simulink model "sbm65_kin"  (R2016b)
settings: Solver=ode45  StartTime=0.0  StopTime=150  MaxStep=.01  RelTol=1e-6  EnableMultiTasking=on
values from neighbouring files (symbols this model uses):
  angFormation1 = 0    [start.m]
  angFormation2 = deg2rad(-45)    [start.m]
  angFormation3 = deg2rad(45)    [start.m]
  deg = pi/180    (= 0.0174532925199)    [db_droni.m]    (also in temp.mat; tslip1.m)
  Di = -77    [start.m]    (also in temp.mat = -77.0888961142)
  ka = 5    [start.m]
  kb = (2/pi*kp - ka + 0.1)*3/5    (= -2.74901406829)    [start.m]
  kp = 0.5    [start.m]
  mis = [  50,   0,   0,  10 ... (first row only)    [start.m]    (also in tslip1.m = [0 0 0)
  wind =     [temp.mat]
  X =     [temp.mat]    (also in tslip1.m = [X [u;eig(AB(1:2,1:2))]])
  X6_ini1 = [2 0   0 0 0 0]'    [start.m]
  X6_ini2 = [  0   0   0 0 0 0]'    [start.m]
  X6_ini3 = [  0  0   0 0 0 0]'    [start.m]
  X7_ini1 = [40 0 -77 1 0 0 0]'    [start.m]
  X7_ini2 = [30 -10 -77 1 0 0 0]'    [start.m]
  X7_ini3 = [20 10 -77 1 0 0 0]'    [start.m]
  xmax = 115    [start.m]
  xmin = -150    [start.m]
  ymax = 105    [start.m]
  ymin = -120    [start.m]
undefined symbols (not defined in the file or in its folder): magnitude, sfunxy2
libraries: simulink x3
settings Model: Creator=hdsvieira  LastModifiedBy=Pedro
settings SolverCC: MaxOrder=2
settings DataIOCC: LimitDataPoints=on  SaveFormat=Array  SignalLoggingSaveFormat=ModelDataLogs  SaveOutput=off  SaveTime=off  SignalLoggingName=sigsOut
settings OptimizationCC: LifeSpan=inf
settings DebuggingCC: ReadBeforeWriteMsg=DisableAll  WriteAfterWriteMsg=DisableAll  WriteAfterReadMsg=DisableAll  SaveWithParameterizedLinksMsg=none  MultiTaskDSMMsg=none  MultiTaskCondExecSysMsg=none  SFUnexpectedBacktrackingDiag=warning  SFNoUnconditionalDefaultTransitionDiag=warning  SFExecutionAtInitializationDiag=none
settings HardwareCC: ProdBitPerPointer=32  ProdBitPerSizeT=32  ProdBitPerPtrDiffT=32  ProdLargestAtomicFloat=None  ProdIntDivRoundTo=Undefined  ProdEndianess=Unspecified  ProdWordSize=32  ProdHWDeviceType=32-bit Generic  TargetUnknown=on
settings ModelReferenceCC: UpdateModelReferenceTargets=IfOutOfDate  PropagateSignalLabelsOutOfModel=off
settings SFSimCC: SFSimEcho=off
settings GRTTargetCC: TargetLangStandard=C89/C90 (ANSI)  GeneratePreprocessorConditionals=Disable all  CombineOutputUpdateFcns=off  GRTInterface=on
settings ConfigComp: CovMetricSettings=dw  CovHtmlReporting=on  CovSaveCumulativeToWorkspaceVar=on  CovSaveSingleToWorkspaceVar=on  CovExternalEMLEnable=off

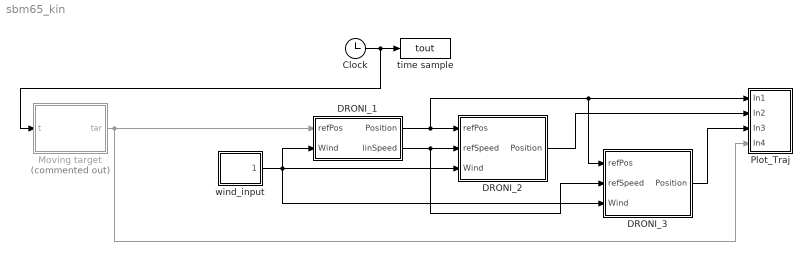
== system sbm65_kin ==
  Clock : Clock
  DRONI_1 : Subsystem
  DRONI_2 : Subsystem
  DRONI_3 : Subsystem
  Moving target : MATLAB Function  Commented=on  TreatAsAtomicUnit=on
  Plot_Traj : Subsystem  LoadFcn=sfunxy2([],[],[],'LoadBlock')  StartFcn=sfunxy2([],[],[],'Start')  StopFcn=sfunxy2([],[],[],'Stop')
      settings: CopyFcn=sfunxy2([],[],[],'CopyBlock')  DeleteFcn=sfunxy2([],[],[],'DeleteBlock')  NameChangeFcn=sfunxy2([],[],[],'NameChange')
  time sample : ToWorkspace  VariableName=tout  SampleTime=X.Toutput
      settings: MaxDataPoints=5000
  wind_input : Subsystem
  wires:
  Clock/1 -> time sample/1, Moving target/1(t)
  DRONI_1/2(linSpeed) -> DRONI_3/2(refSpeed), DRONI_2/2(refSpeed)
  DRONI_3/1(Position) -> Plot_Traj/3(In3)
  DRONI_2/1(Position) -> Plot_Traj/2(In2)
  DRONI_1/1(Position) -> DRONI_3/1(refPos), Plot_Traj/1(In1), DRONI_2/1(refPos)
  Moving target/1(tar) -> DRONI_1/1(refPos), Plot_Traj/4(In4)
  wind_input/1(U_wind) -> DRONI_3/3(Wind), DRONI_1/2(Wind), DRONI_2/3(Wind)

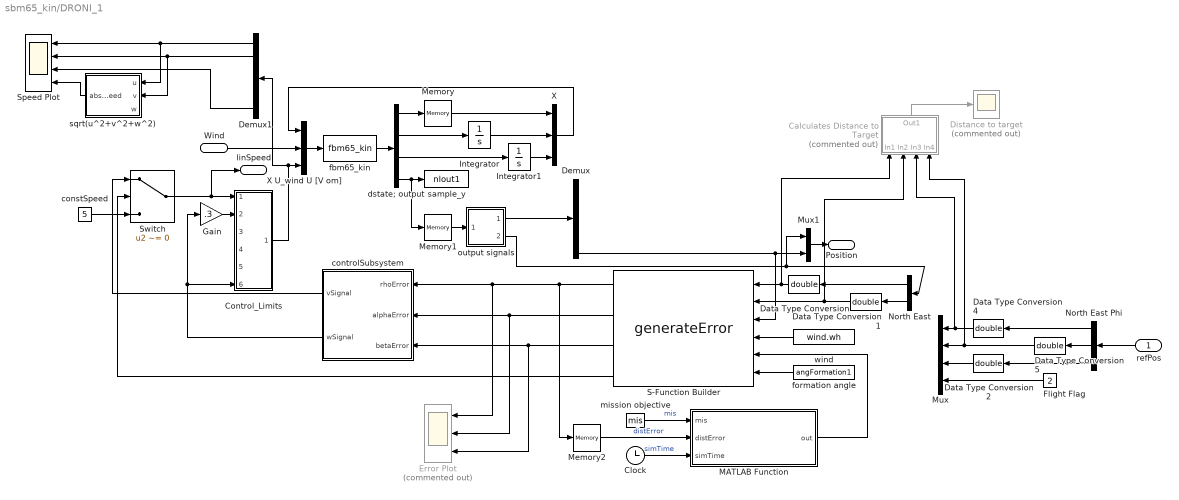
== system sbm65_kin/DRONI_1 ==
  refPos : Inport
  Wind : Inport  Port=2
  Calculates Distance to Target : Subsystem  Commented=on
  Clock : Clock
  Control_Limits : Subsystem
  Data Type Conversion{,1..2,4..5} (5 alike) : DataTypeConversion  DisableCoverage=on  OutDataTypeStr=double
  Demux : Demux  Outputs=5
  Demux1 : Demux  Outputs=6
  Distance to target : Scope  Commented=on
  Error Plot : Scope  Commented=on  NumInputPorts=3
  Flight Flag : Constant  Value=2
  Gain : Gain  Gain=.3
  Integrator : Integrator  InitialCondition=X7_ini1
  Integrator1 : Integrator  InitialCondition=zeros(1,8)
  MATLAB Function : MATLAB Function  TreatAsAtomicUnit=on
  Memory : Memory  X0=X6_ini1
  Memory1 : Memory  X0=zeros(22,1)
  Memory2 : Memory  X0=10
  Mux : Mux
  Mux1 : Mux  Inputs=2
  North East : Demux  Outputs=[1 1]
  North East Phi : Demux  Outputs=[1 1 1]
  S-Function Builder : S-Function  InitFcn=try, set_param(gcb,'FunctionName','generateError'), end  FunctionName=generateError  SFunctionModules=generateError_wrapper  SFunctionDeploymentMode=off  EnableBusSupport=off  mask(S-Function Builder){}
      mask help: Simulink:masks:SFunctionBuilder_MD
      mask init:
      | val = [[.9  0.75 0.75 1 1 .9 .9 1]',[1 1 0.75 0.75 .9 .9 1 .9]'];try , sys = get_param(gcb,'SfunBuilderFcnName');if isempty(sys), sys = get_param(gcb,'FunctionName'); end,catch, sys = get_param(gcb,'FunctionName'); end
      settings: CopyFcn=set_param(gcbh,'LinkStatus','none')  PreSaveFcn=try, set_param(gcb,'FunctionName','generateError'), end  OpenFcn=sfunctionwizard(gcbh)
      mask Display: plot(val(:,1),val(:,2)),disp(sys), port_label('input',1,'y0'), port_label('input',2,'x0'), port_label('input',3,'theta0'), port_label('input',4,'wind'), port_label('input',5,'objective'), port_label('input',6,'angOffset'), port_label('output',1,'rho'), port_label('output',2,'alpha'), port_label('output',3,'beta'), port_label('output',4,'flightMode')
  Speed Plot : Scope  NumInputPorts=4
  Switch : Switch  Criteria=u2 ~= 0  Threshold=.5
  X : Mux  Inputs=[6 7 8]
  X U_wind U [V om] : Mux  Inputs=[21 5 6]
  constSpeed : Constant  Value=5
  controlSubsystem : Subsystem
  dstate; output : Demux  Outputs="[6 7  8  22]"
  fbm65_kin : MATLABFcn  MATLABFcn=fbm65_kin  OutputDimensions=43
  formation angle : Constant  Value=angFormation1
  mission objective : Constant  Value=mis
  output signals : Subsystem
  sample_y : ToWorkspace  VariableName=nlout1  SampleTime=X.Toutput
      settings: MaxDataPoints=5000
  sqrt(u^2+v^2+w^2) : Subsystem
  wind : Constant  Value=wind.wh
  Position : Outport
  linSpeed : Outport  Port=2
  wires:
  North East/2 -> Data Type Conversion1/1
  Memory1/1 -> output signals/1(nlout)
  X U_wind U [V om]/1 -> fbm65_kin/1
  fbm65_kin/1 -> dstate; output/1
  Control_Limits/1(Out1) -> Demux1/1, X U_wind U [V om]/3
  dstate; output/3 -> Integrator1/1
  Integrator/1 -> X/2
  wind/1 -> S-Function Builder/4
  Integrator1/1 -> X/3
  dstate; output/1 -> Memory/1
  Memory/1 -> X/1
  Data Type Conversion/1 -> S-Function Builder/1, Calculates Distance to Target/1(In1)
  North East/1 -> Data Type Conversion/1
  dstate; output/2 -> Integrator/1
  output signals/1(Out1) -> Demux/1
  X/1 -> X U_wind U [V om]/1
  Data Type Conversion1/1 -> S-Function Builder/2, Calculates Distance to Target/2(In2)
  Wind/1 -> X U_wind U [V om]/2
  controlSubsystem/2(wSignal) -> Control_Limits/6(In6), Gain/1
  Switch/1 -> linSpeed/1, Control_Limits/1(In1)
  S-Function Builder/4 -> Switch/2
  constSpeed/1 -> Switch/3
  controlSubsystem/1(vSignal) -> Switch/1
  dstate; output/4 -> sample_y/1, Memory1/1
  Demux/5 -> Mux1/2, S-Function Builder/3
  output signals/2(Out2) -> Mux1/1, North East/1
  S-Function Builder/1 -> Memory2/1, Error Plot/1, controlSubsystem/1(rhoError)
  S-Function Builder/2 -> Error Plot/2, controlSubsystem/2(alphaError)
  S-Function Builder/3 -> Error Plot/3, controlSubsystem/3(betaError)
  Clock/1 -> MATLAB Function/3(simTime)  "simTime"
  Memory2/1 -> MATLAB Function/2(distError)  "distError"
  mission objective/1 -> MATLAB Function/1(mis)  "mis"
  Demux1/1 -> Speed Plot/1, sqrt(u^2+v^2+w^2)/1(u)
  Demux1/2 -> sqrt(u^2+v^2+w^2)/2(v), Speed Plot/2
  sqrt(u^2+v^2+w^2)/1(abs speed) -> Speed Plot/4
  Gain/1 -> Control_Limits/2(In2)
  North East Phi/2 -> Data Type Conversion5/1
  North East Phi/1 -> Data Type Conversion4/1
  refPos/1 -> North East Phi/1
  North East Phi/3 -> Data Type Conversion2/1
  Data Type Conversion4/1 -> Calculates Distance to Target/3(In3), Mux/1
  Data Type Conversion5/1 -> Calculates Distance to Target/4(In4), Mux/2
  Data Type Conversion2/1 -> Mux/3
  Flight Flag/1 -> Mux/4
  formation angle/1 -> S-Function Builder/6
  Mux1/1 -> Position/1
  Demux1/6 -> Speed Plot/3
  Calculates Distance to Target/1(Out1) -> Distance to target/1
  MATLAB Function/1(out) -> S-Function Builder/5

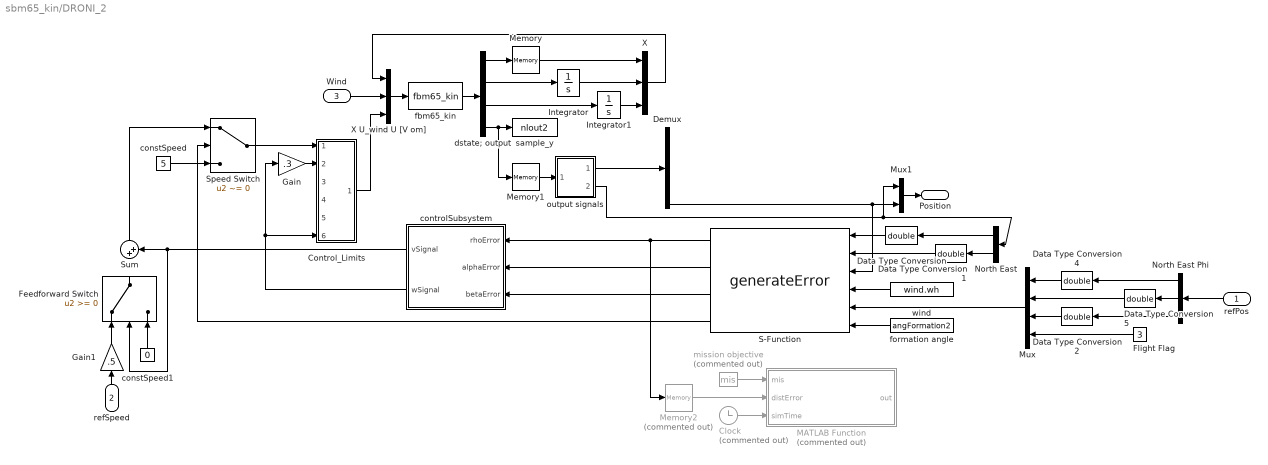
== system sbm65_kin/DRONI_2 ==
  refPos : Inport
  refSpeed : Inport  Port=2
  Wind : Inport  Port=3
  Clock : Clock  Commented=on
  Control_Limits : Subsystem
  Data Type Conversion{,1..2,4..5} (5 alike) : DataTypeConversion  DisableCoverage=on  OutDataTypeStr=double
  Demux : Demux  Outputs=5
  Feedforward Switch : Switch
  Flight Flag : Constant  Value=3
  Gain : Gain  Gain=.3
  Gain1 : Gain  Gain=.5
  Integrator : Integrator  InitialCondition=X7_ini2
  Integrator1 : Integrator  InitialCondition=zeros(1,8)
  MATLAB Function : MATLAB Function  Commented=on  TreatAsAtomicUnit=on
  Memory : Memory  X0=X6_ini2
  Memory1 : Memory  X0=zeros(22,1)
  Memory2 : Memory  Commented=on  X0=10
  Mux : Mux
  Mux1 : Mux  Inputs=2
  North East : Demux  Outputs=[1 1]
  North East Phi : Demux  Outputs=[1 1 1]
  S-Function : S-Function  FunctionName=generateError  SFunctionDeploymentMode=off  EnableBusSupport=off
  Speed Switch : Switch  Criteria=u2 ~= 0  Threshold=.5
  Sum : Sum  Inputs=|++
  X : Mux  Inputs=[6 7 8]
  X U_wind U [V om] : Mux  Inputs=[21 5 6]
  constSpeed : Constant  Value=5
  constSpeed1 : Constant  Value=0
  controlSubsystem : Subsystem
  dstate; output : Demux  Outputs="[6 7  8  22]"
  fbm65_kin : MATLABFcn  MATLABFcn=fbm65_kin  OutputDimensions=43
  formation angle : Constant  Value=angFormation2
  mission objective : Constant  Commented=on  Value=mis
  output signals : Subsystem
  sample_y : ToWorkspace  VariableName=nlout2  SampleTime=X.Toutput
      settings: MaxDataPoints=5000
  wind : Constant  Value=wind.wh
  Position : Outport
  wires:
  North East/2 -> Data Type Conversion1/1
  Memory1/1 -> output signals/1(nlout)
  X U_wind U [V om]/1 -> fbm65_kin/1
  fbm65_kin/1 -> dstate; output/1
  Control_Limits/1(Out1) -> X U_wind U [V om]/3
  dstate; output/3 -> Integrator1/1
  Integrator/1 -> X/2
  wind/1 -> S-Function/4
  Integrator1/1 -> X/3
  dstate; output/1 -> Memory/1
  Memory/1 -> X/1
  Data Type Conversion/1 -> S-Function/1
  North East/1 -> Data Type Conversion/1
  dstate; output/2 -> Integrator/1
  output signals/1(Out1) -> Demux/1
  X/1 -> X U_wind U [V om]/1
  Data Type Conversion1/1 -> S-Function/2
  Wind/1 -> X U_wind U [V om]/2
  mission objective/1 -> MATLAB Function/1(mis)
  Clock/1 -> MATLAB Function/3(simTime)
  Memory2/1 -> MATLAB Function/2(distError)
  Speed Switch/1 -> Control_Limits/1(In1)
  S-Function/4 -> Speed Switch/2
  constSpeed/1 -> Speed Switch/3
  controlSubsystem/1(vSignal) -> Feedforward Switch/2, Sum/2
  dstate; output/4 -> sample_y/1, Memory1/1
  Demux/5 -> Mux1/2, S-Function/3
  output signals/2(Out2) -> Mux1/1, North East/1
  S-Function/1 -> Memory2/1, controlSubsystem/1(rhoError)
  S-Function/2 -> controlSubsystem/2(alphaError)
  S-Function/3 -> controlSubsystem/3(betaError)
  Data Type Conversion4/1 -> Mux/1
  Data Type Conversion5/1 -> Mux/2
  Data Type Conversion2/1 -> Mux/3
  Mux/1 -> S-Function/5
  Flight Flag/1 -> Mux/4
  formation angle/1 -> S-Function/6
  Sum/1 -> Speed Switch/1
  controlSubsystem/2(wSignal) -> Control_Limits/6(In6), Gain/1
  refSpeed/1 -> Gain1/1
  Gain/1 -> Control_Limits/2(In2)
  North East Phi/2 -> Data Type Conversion5/1
  North East Phi/1 -> Data Type Conversion4/1
  refPos/1 -> North East Phi/1
  North East Phi/3 -> Data Type Conversion2/1
  Mux1/1 -> Position/1
  Gain1/1 -> Feedforward Switch/1
  constSpeed1/1 -> Feedforward Switch/3

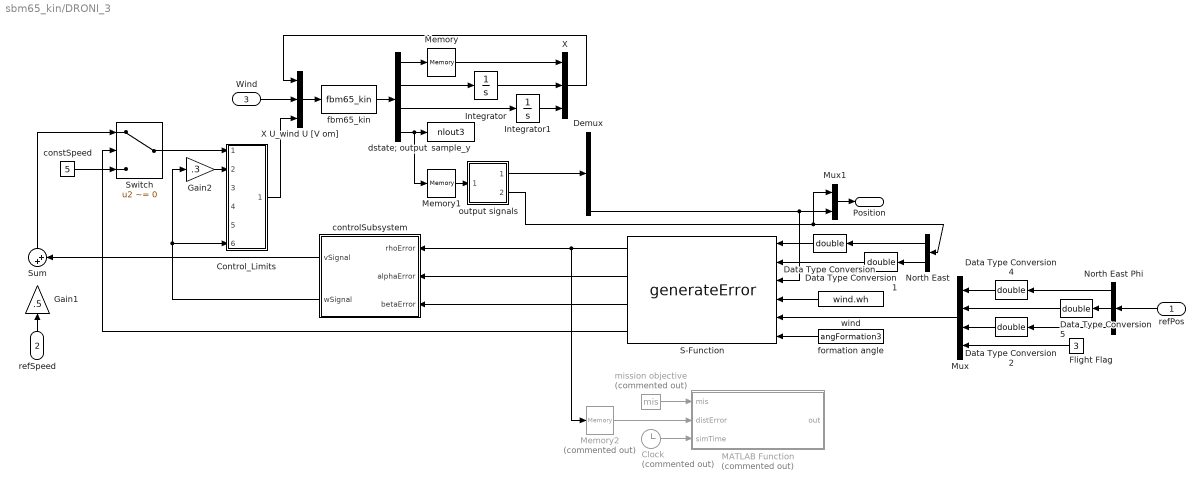
== system sbm65_kin/DRONI_3 ==
  refPos : Inport
  refSpeed : Inport  Port=2
  Wind : Inport  Port=3
  Clock : Clock  Commented=on
  Control_Limits : Subsystem
  Data Type Conversion{,1..2,4..5} (5 alike) : DataTypeConversion  DisableCoverage=on  OutDataTypeStr=double
  Demux : Demux  Outputs=5
  Flight Flag : Constant  Value=3
  Gain1 : Gain  Gain=.5
  Gain2 : Gain  Gain=.3
  Integrator : Integrator  InitialCondition=X7_ini3
  Integrator1 : Integrator  InitialCondition=zeros(1,8)
  MATLAB Function : MATLAB Function  Commented=on  TreatAsAtomicUnit=on
  Memory : Memory  X0=X6_ini3
  Memory1 : Memory  X0=zeros(22,1)
  Memory2 : Memory  Commented=on  X0=10
  Mux : Mux
  Mux1 : Mux  Inputs=2
  North East : Demux  Outputs=[1 1]
  North East Phi : Demux  Outputs=[1 1 1]
  S-Function : S-Function  FunctionName=generateError  SFunctionDeploymentMode=off  EnableBusSupport=off
  Sum : Sum  Inputs=|++
  Switch : Switch  Criteria=u2 ~= 0  Threshold=.5
  X : Mux  Inputs=[6 7 8]
  X U_wind U [V om] : Mux  Inputs=[21 5 6]
  constSpeed : Constant  Value=5
  controlSubsystem : Subsystem
  dstate; output : Demux  Outputs="[6 7  8  22]"
  fbm65_kin : MATLABFcn  MATLABFcn=fbm65_kin  OutputDimensions=43
  formation angle : Constant  Value=angFormation3
  mission objective : Constant  Commented=on  Value=mis
  output signals : Subsystem
  sample_y : ToWorkspace  VariableName=nlout3  SampleTime=X.Toutput
      settings: MaxDataPoints=5000
  wind : Constant  Value=wind.wh
  Position : Outport
  wires:
  North East/2 -> Data Type Conversion1/1
  Memory1/1 -> output signals/1(nlout)
  X U_wind U [V om]/1 -> fbm65_kin/1
  fbm65_kin/1 -> dstate; output/1
  Control_Limits/1(Out1) -> X U_wind U [V om]/3
  dstate; output/3 -> Integrator1/1
  Integrator/1 -> X/2
  wind/1 -> S-Function/4
  Integrator1/1 -> X/3
  dstate; output/1 -> Memory/1
  Memory/1 -> X/1
  Data Type Conversion/1 -> S-Function/1
  North East/1 -> Data Type Conversion/1
  dstate; output/2 -> Integrator/1
  output signals/1(Out1) -> Demux/1
  X/1 -> X U_wind U [V om]/1
  Data Type Conversion1/1 -> S-Function/2
  Wind/1 -> X U_wind U [V om]/2
  mission objective/1 -> MATLAB Function/1(mis)
  Clock/1 -> MATLAB Function/3(simTime)
  controlSubsystem/2(wSignal) -> Control_Limits/6(In6), Gain2/1
  Memory2/1 -> MATLAB Function/2(distError)
  S-Function/4 -> Switch/2
  constSpeed/1 -> Switch/3
  dstate; output/4 -> sample_y/1, Memory1/1
  Demux/5 -> Mux1/2, S-Function/3
  output signals/2(Out2) -> Mux1/1, North East/1
  S-Function/1 -> Memory2/1, controlSubsystem/1(rhoError)
  S-Function/2 -> controlSubsystem/2(alphaError)
  S-Function/3 -> controlSubsystem/3(betaError)
  Data Type Conversion4/1 -> Mux/1
  Data Type Conversion5/1 -> Mux/2
  Data Type Conversion2/1 -> Mux/3
  Mux/1 -> S-Function/5
  Flight Flag/1 -> Mux/4
  formation angle/1 -> S-Function/6
  controlSubsystem/1(vSignal) -> Sum/2
  Sum/1 -> Switch/1
  refSpeed/1 -> Gain1/1
  Mux1/1 -> Position/1
  North East Phi/2 -> Data Type Conversion5/1
  North East Phi/1 -> Data Type Conversion4/1
  refPos/1 -> North East Phi/1
  North East Phi/3 -> Data Type Conversion2/1
  Gain2/1 -> Control_Limits/2(In2)
  Switch/1 -> Control_Limits/1(In1)

== system sbm65_kin/Plot_Traj ==
  In1 : Inport
  In2 : Inport  Port=2
  In3 : Inport  Port=3
  In4 : Inport  Port=4
  Mux : Mux
  Mux1 : Mux  Inputs=8
  Subsystem : Subsystem
  To Workspace : ToWorkspace  VariableName=trajectories  SampleTime=-1
  sfunxy : S-Function  Commented=on  DisableCoverage=on  FunctionName=sfunxy2  Parameters=[xmin xmax ymin ymax], autoscale  SFunctionDeploymentMode=off  EnableBusSupport=off  mask(XY Scope (Custom)){xmin=xmin, xmax=xmax, ymin=ymin, ymax=ymax, autoscale=off}
      mask prompts: xmin "X-min"; xmax "X-max"; ymin "Y-min"; ymax "Y-max"; autoscale "Graph Autoscale"
      mask help: Plots second input (Y) against first input (X) at each time step to create an X-Y plot. Ignores data outside the ranges specified by x-min, x-max, y-min, y-max.
      mask Help: This block can be used to explore limit cycles. Look at the m-file sfunxy.m to see how it works.
      mask Display: plot([.05 .95 .95 .05 .05],[.45 .45 .95 .95 .45], 0.5+cos(0:0.1:2*pi)*0.3,0.7+sin(0:0.1:2*pi)*0.2)
  wires:
  In2/1 -> Subsystem/2(In2)
  Mux1/1 -> To Workspace/1
  In3/1 -> Subsystem/3(In3)
  Mux/1 -> sfunxy/1
  In1/1 -> Subsystem/1(In1)
  In4/1 -> Subsystem/4(In4)
  Subsystem/2(Out2) -> Mux1/2
  Subsystem/4(Out4) -> Mux1/4
  Subsystem/6(Out6) -> Mux1/6
  Subsystem/8(Out8) -> Mux1/8
  Subsystem/7(Out7) -> Mux1/7, Mux/4
  Subsystem/5(Out5) -> Mux1/5, Mux/3
  Subsystem/3(Out3) -> Mux1/3, Mux/2
  Subsystem/1(Out1) -> Mux1/1, Mux/1

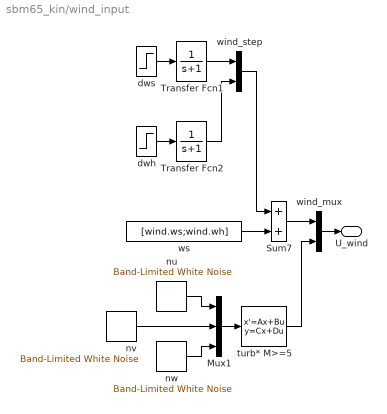
== system sbm65_kin/wind_input ==
  Mux1 : Mux  Inputs=3
  Sum7 : Sum  SaturateOnIntegerOverflow=on  InputSameDT=on  OutDataTypeStr=Inherit: Same as first input
  Transfer Fcn1 : TransferFcn  Denominator=[1 1]
  Transfer Fcn2 : TransferFcn  Denominator=[1 1]
  dwh : Step  Time=wind.tws  After=wind.dwh  SampleTime=0
  dws : Step  Time=wind.tws  After=wind.dws  SampleTime=0
  nu : simulink/Sources/Band-Limited White Noise  Cov=wind.Tsw/2  Ts=wind.Tsw/2  seed=[23341]
  nv : simulink/Sources/Band-Limited White Noise  Cov=wind.Tsw/2  Ts=wind.Tsw/2  seed=[2334]
  nw : simulink/Sources/Band-Limited White Noise  Cov=wind.Tsw/2  Ts=wind.Tsw/2  seed=[233]
  turb* M>=5 : StateSpace  A=[]  B=[]  C=[]  D=K  X0=0  mask(K){K=eye(3)*wind.sigg*wind.turb}
      mask prompts: K "K="
      mask help: Matrix gain
      mask Display: disp('K')
  wind_mux : Mux  Inputs=[2 3]
  wind_step : Mux  Inputs=2
  ws : Constant  Value=[wind.ws;wind.wh]
  U_wind : Outport
  wires:
  Mux1/1 -> turb* M>=5/1
  dwh/1 -> Transfer Fcn2/1
  wind_mux/1 -> U_wind/1
  dws/1 -> Transfer Fcn1/1
  Transfer Fcn1/1 -> wind_step/1
  ws/1 -> Sum7/2
  Sum7/1 -> wind_mux/1
  nw/1 -> Mux1/3
  nu/1 -> Mux1/1
  nv/1 -> Mux1/2
  Transfer Fcn2/1 -> wind_step/2
  turb* M>=5/1 -> wind_mux/2
  wind_step/1 -> Sum7/1

== system sbm65_kin/DRONI_1/Calculates Distance to Target ==
  In1 : Inport
  In2 : Inport  Port=2
  In3 : Inport  Port=3
  In4 : Inport  Port=4
  Product : Product
  Product1 : Product
  Sqrt : Sqrt  SaturateOnIntegerOverflow=on
  Sum : Sum  Inputs=+-
  Sum1 : Sum  Inputs=+-
  Sum2 : Sum
  Out1 : Outport
  wires:
  Product/1 -> Sum2/1
  Sum2/1 -> Sqrt/1
  Sum1/1 -> Product1/1, Product1/2
  Sqrt/1 -> Out1/1
  In1/1 -> Sum/1
  In2/1 -> Sum1/1
  In4/1 -> Sum1/2
  In3/1 -> Sum/2
  Sum/1 -> Product/1, Product/2
  Product1/1 -> Sum2/2

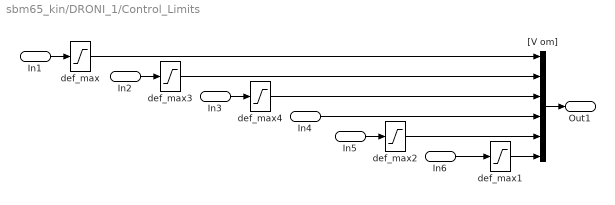
== system sbm65_kin/DRONI_1/Control_Limits ==
  In1 : Inport
  In2 : Inport  Port=2
  In3 : Inport  Port=3
  In4 : Inport  Port=4
  In5 : Inport  Port=5
  In6 : Inport  Port=6
  "[V om]" : Mux  Inputs=[1 1 1 1 1 1]
  def_max : Saturate  UpperLimit=9  LowerLimit=0
  def_max1 : Saturate  UpperLimit=20*deg  LowerLimit=-20*deg
  def_max2 : Saturate  UpperLimit=20*deg  LowerLimit=-20*deg
  def_max3 : Saturate  UpperLimit=1  LowerLimit=-1
  def_max4 : Saturate  UpperLimit=10  LowerLimit=-10
  Out1 : Outport
  wires:
  In6/1 -> def_max1/1
  "[V om]"/1 -> Out1/1
  In2/1 -> def_max3/1
  In1/1 -> def_max/1
  In5/1 -> def_max2/1
  def_max1/1 -> "[V om]"/6
  In3/1 -> def_max4/1
  def_max2/1 -> "[V om]"/5
  In4/1 -> "[V om]"/4
  def_max4/1 -> "[V om]"/3
  def_max3/1 -> "[V om]"/2
  def_max/1 -> "[V om]"/1

== system sbm65_kin/DRONI_1/controlSubsystem ==
  rhoError : Inport
  alphaError : Inport  Port=2
  betaError : Inport  Port=3
  Gain : Gain  Gain=kp
  Gain1 : Gain  Gain=ka
  Gain2 : Gain  Gain=kb
  Sum : Sum  Inputs=|++
  vSignal : Outport
  wSignal : Outport  Port=2
  wires:
  Gain/1 -> vSignal/1
  betaError/1 -> Gain2/1
  Sum/1 -> wSignal/1
  Gain1/1 -> Sum/1
  alphaError/1 -> Gain1/1
  rhoError/1 -> Gain/1
  Gain2/1 -> Sum/2

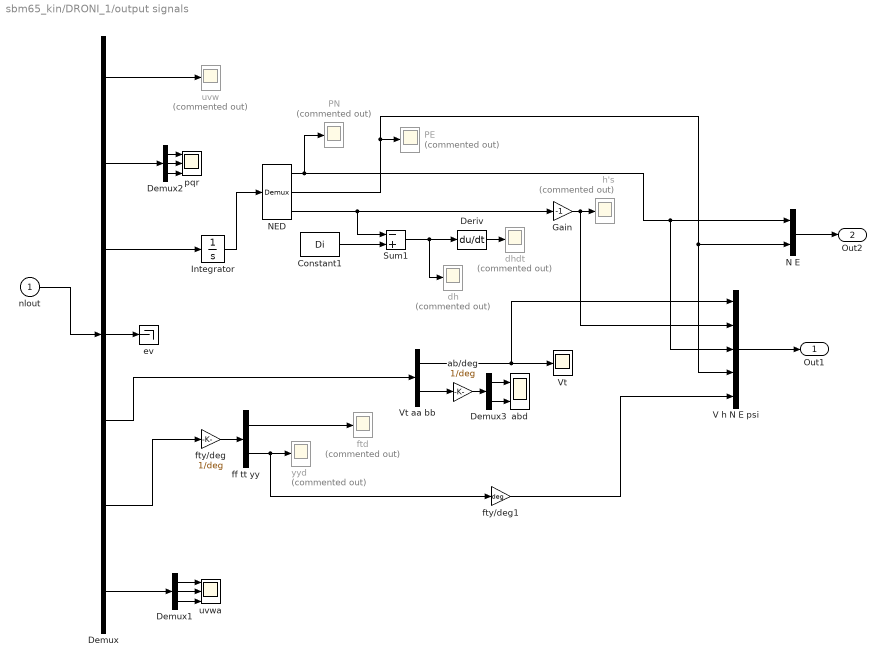
== system sbm65_kin/DRONI_1/output signals ==
  nlout : Inport
  Constant1 : Constant  Value=Di
  Demux : Demux  Outputs=[3 3 3 4 3 3 3]
  Demux1 : Demux  Outputs=3
  Demux2 : Demux  Outputs=3
  Demux3 : Demux  Outputs=2
  Deriv : Derivative
  Gain : Gain  Gain=-1  SaturateOnIntegerOverflow=on  OutDataTypeStr=Inherit: Same as input  ParamDataTypeStr=Inherit: Same as input
  Integrator : Integrator  InitialCondition=X7_ini1(1:3)
  N E : Mux  Inputs=2
  NED : Demux  Outputs=3
  PE : Scope  Commented=on
  PN : Scope  Commented=on
  Sum1 : Sum  Inputs=-+  SaturateOnIntegerOverflow=on  InputSameDT=on  OutDataTypeStr=Inherit: Same as first input
  V h N E psi : Mux  Inputs=5
  Vt : Scope
  Vt aa bb : Demux  Outputs=[1 2]
  ab/deg : Gain  Gain=1/deg  SaturateOnIntegerOverflow=on  OutDataTypeStr=Inherit: Same as input  ParamDataTypeStr=Inherit: Same as input
  abd : Scope  NumInputPorts=2
  dh : Scope  Commented=on
  dhdt : Scope  Commented=on
  ev : Terminator
  ff tt yy : Demux  Outputs=[2 1]
  ftd : Scope  Commented=on
  fty/deg : Gain  Gain=1/deg  SaturateOnIntegerOverflow=on  OutDataTypeStr=Inherit: Same as input  ParamDataTypeStr=Inherit: Same as input
  fty/deg1 : Gain  Gain=deg  SaturateOnIntegerOverflow=on  OutDataTypeStr=Inherit: Same as input  ParamDataTypeStr=Inherit: Same as input
  h's : Scope  Commented=on
  pqr : Scope  NumInputPorts=3
  uvw : Scope  Commented=on
  uvwa : Scope  NumInputPorts=3
  yyd : Scope  Commented=on
  Out1 : Outport
  Out2 : Outport  Port=2
  wires:
  fty/deg/1 -> ff tt yy/1
  NED/1 -> PN/1, N E/1, V h N E psi/3
  NED/2 -> PE/1, N E/2, V h N E psi/4
  Gain/1 -> V h N E psi/2, h's/1
  NED/3 -> Gain/1, Sum1/1
  Sum1/1 -> dh/1, Deriv/1
  Constant1/1 -> Sum1/2
  Demux/4 -> ev/1
  Vt aa bb/2 -> ab/deg/1
  Vt aa bb/1 -> V h N E psi/1, Vt/1
  nlout/1 -> Demux/1
  ff tt yy/1 -> ftd/1
  ff tt yy/2 -> fty/deg1/1, yyd/1
  Deriv/1 -> dhdt/1
  Demux/1 -> uvw/1
  Demux/3 -> Integrator/1
  Demux/5 -> Vt aa bb/1
  Demux/6 -> fty/deg/1
  Integrator/1 -> NED/1
  fty/deg1/1 -> V h N E psi/5
  V h N E psi/1 -> Out1/1
  N E/1 -> Out2/1
  Demux1/1 -> uvwa/1
  Demux1/2 -> uvwa/2
  Demux1/3 -> uvwa/3
  Demux/7 -> Demux1/1
  Demux2/1 -> pqr/1
  Demux2/2 -> pqr/2
  Demux2/3 -> pqr/3
  Demux/2 -> Demux2/1
  ab/deg/1 -> Demux3/1
  Demux3/1 -> abd/1
  Demux3/2 -> abd/2

== system sbm65_kin/DRONI_1/sqrt(u^2+v^2+w^2) ==
  u : Inport
  v : Inport  Port=2
  w : Inport  Port=3
  Math Function : Math  Operator=magnitude^2  OutputSignalType=real  SaturateOnIntegerOverflow=on
  Math Function1 : Math  Operator=magnitude^2  OutputSignalType=real  SaturateOnIntegerOverflow=on
  Math Function2 : Math  Operator=magnitude^2  OutputSignalType=real  SaturateOnIntegerOverflow=on
  Sqrt : Sqrt  SaturateOnIntegerOverflow=on
  Sum of Elements : Sum  Inputs=+++
  abs speed : Outport
  wires:
  Sum of Elements/1 -> Sqrt/1
  Sqrt/1 -> abs speed/1
  v/1 -> Math Function1/1
  u/1 -> Math Function/1
  w/1 -> Math Function2/1
  Math Function1/1 -> Sum of Elements/2
  Math Function2/1 -> Sum of Elements/3
  Math Function/1 -> Sum of Elements/1

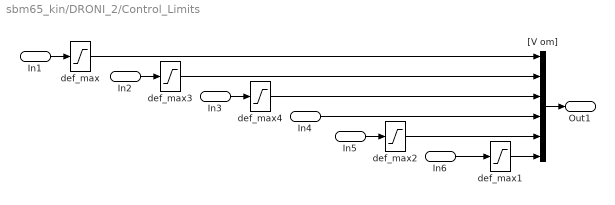
== system sbm65_kin/DRONI_2/Control_Limits ==
  In1 : Inport
  In2 : Inport  Port=2
  In3 : Inport  Port=3
  In4 : Inport  Port=4
  In5 : Inport  Port=5
  In6 : Inport  Port=6
  "[V om]" : Mux  Inputs=[1 1 1 1 1 1]
  def_max : Saturate  UpperLimit=9  LowerLimit=0
  def_max1 : Saturate  UpperLimit=20*deg  LowerLimit=-20*deg
  def_max2 : Saturate  UpperLimit=20*deg  LowerLimit=-20*deg
  def_max3 : Saturate  UpperLimit=1  LowerLimit=-1
  def_max4 : Saturate  UpperLimit=10  LowerLimit=-10
  Out1 : Outport
  wires:
  In6/1 -> def_max1/1
  "[V om]"/1 -> Out1/1
  In2/1 -> def_max3/1
  In1/1 -> def_max/1
  In5/1 -> def_max2/1
  def_max1/1 -> "[V om]"/6
  In3/1 -> def_max4/1
  def_max2/1 -> "[V om]"/5
  In4/1 -> "[V om]"/4
  def_max4/1 -> "[V om]"/3
  def_max3/1 -> "[V om]"/2
  def_max/1 -> "[V om]"/1

== system sbm65_kin/DRONI_2/controlSubsystem ==
  rhoError : Inport
  alphaError : Inport  Port=2
  betaError : Inport  Port=3
  Gain : Gain  Gain=kp
  Gain1 : Gain  Gain=ka
  Gain2 : Gain  Gain=kb
  Sum : Sum  Inputs=|++
  vSignal : Outport
  wSignal : Outport  Port=2
  wires:
  Gain/1 -> vSignal/1
  betaError/1 -> Gain2/1
  Sum/1 -> wSignal/1
  Gain1/1 -> Sum/1
  alphaError/1 -> Gain1/1
  rhoError/1 -> Gain/1
  Gain2/1 -> Sum/2

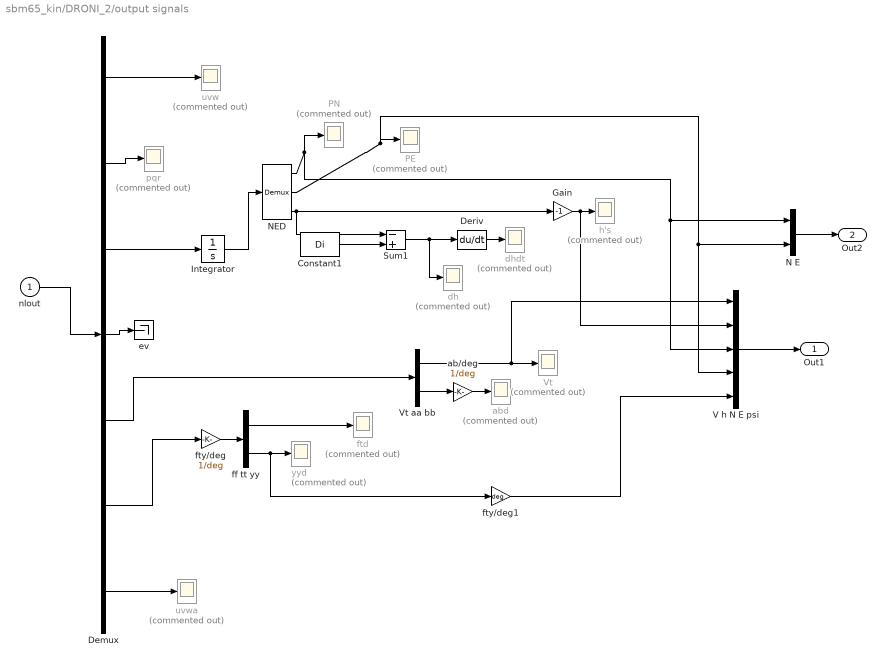
== system sbm65_kin/DRONI_2/output signals ==
  nlout : Inport
  Constant1 : Constant  Value=Di
  Demux : Demux  Outputs=[3 3 3 4 3 3 3]
  Deriv : Derivative
  Gain : Gain  Gain=-1  SaturateOnIntegerOverflow=on  OutDataTypeStr=Inherit: Same as input  ParamDataTypeStr=Inherit: Same as input
  Integrator : Integrator  InitialCondition=X7_ini2(1:3)
  N E : Mux  Inputs=2
  NED : Demux  Outputs=3
  PE : Scope  Commented=on
  PN : Scope  Commented=on
  Sum1 : Sum  Inputs=-+  SaturateOnIntegerOverflow=on  InputSameDT=on  OutDataTypeStr=Inherit: Same as first input
  V h N E psi : Mux  Inputs=5
  Vt : Scope  Commented=on
  Vt aa bb : Demux  Outputs=[1 2]
  ab/deg : Gain  Gain=1/deg  SaturateOnIntegerOverflow=on  OutDataTypeStr=Inherit: Same as input  ParamDataTypeStr=Inherit: Same as input
  abd : Scope  Commented=on
  dh : Scope  Commented=on
  dhdt : Scope  Commented=on
  ev : Terminator
  ff tt yy : Demux  Outputs=[2 1]
  ftd : Scope  Commented=on
  fty/deg : Gain  Gain=1/deg  SaturateOnIntegerOverflow=on  OutDataTypeStr=Inherit: Same as input  ParamDataTypeStr=Inherit: Same as input
  fty/deg1 : Gain  Gain=deg  SaturateOnIntegerOverflow=on  OutDataTypeStr=Inherit: Same as input  ParamDataTypeStr=Inherit: Same as input
  h's : Scope  Commented=on
  pqr : Scope  Commented=on
  uvw : Scope  Commented=on
  uvwa : Scope  Commented=on
  yyd : Scope  Commented=on
  Out1 : Outport
  Out2 : Outport  Port=2
  wires:
  fty/deg/1 -> ff tt yy/1
  ab/deg/1 -> abd/1
  NED/1 -> N E/1, V h N E psi/3, PN/1
  NED/2 -> N E/2, V h N E psi/4, PE/1
  Gain/1 -> V h N E psi/2, h's/1
  NED/3 -> Gain/1, Sum1/1
  Sum1/1 -> dh/1, Deriv/1
  Constant1/1 -> Sum1/2
  Demux/4 -> ev/1
  Vt aa bb/2 -> ab/deg/1
  Vt aa bb/1 -> V h N E psi/1, Vt/1
  nlout/1 -> Demux/1
  Demux/2 -> pqr/1
  ff tt yy/1 -> ftd/1
  ff tt yy/2 -> fty/deg1/1, yyd/1
  Deriv/1 -> dhdt/1
  Demux/1 -> uvw/1
  Demux/3 -> Integrator/1
  Demux/5 -> Vt aa bb/1
  Demux/6 -> fty/deg/1
  Demux/7 -> uvwa/1
  Integrator/1 -> NED/1
  fty/deg1/1 -> V h N E psi/5
  V h N E psi/1 -> Out1/1
  N E/1 -> Out2/1

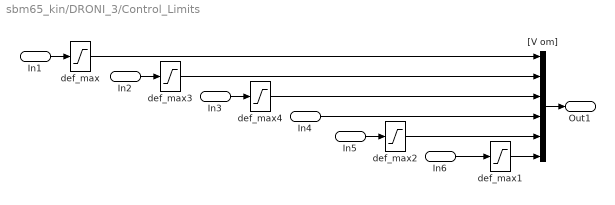
== system sbm65_kin/DRONI_3/Control_Limits ==
  In1 : Inport
  In2 : Inport  Port=2
  In3 : Inport  Port=3
  In4 : Inport  Port=4
  In5 : Inport  Port=5
  In6 : Inport  Port=6
  "[V om]" : Mux  Inputs=[1 1 1 1 1 1]
  def_max : Saturate  UpperLimit=9  LowerLimit=0
  def_max1 : Saturate  UpperLimit=20*deg  LowerLimit=-20*deg
  def_max2 : Saturate  UpperLimit=20*deg  LowerLimit=-20*deg
  def_max3 : Saturate  UpperLimit=1  LowerLimit=-1
  def_max4 : Saturate  UpperLimit=10  LowerLimit=-10
  Out1 : Outport
  wires:
  In6/1 -> def_max1/1
  "[V om]"/1 -> Out1/1
  In2/1 -> def_max3/1
  In1/1 -> def_max/1
  In5/1 -> def_max2/1
  def_max1/1 -> "[V om]"/6
  In3/1 -> def_max4/1
  def_max2/1 -> "[V om]"/5
  In4/1 -> "[V om]"/4
  def_max4/1 -> "[V om]"/3
  def_max3/1 -> "[V om]"/2
  def_max/1 -> "[V om]"/1

== system sbm65_kin/DRONI_3/controlSubsystem ==
  rhoError : Inport
  alphaError : Inport  Port=2
  betaError : Inport  Port=3
  Gain : Gain  Gain=kp
  Gain1 : Gain  Gain=ka
  Gain2 : Gain  Gain=kb
  Sum : Sum  Inputs=|++
  vSignal : Outport
  wSignal : Outport  Port=2
  wires:
  Gain/1 -> vSignal/1
  Sum/1 -> wSignal/1
  alphaError/1 -> Gain1/1
  rhoError/1 -> Gain/1
  Gain2/1 -> Sum/2
  Gain1/1 -> Sum/1
  betaError/1 -> Gain2/1

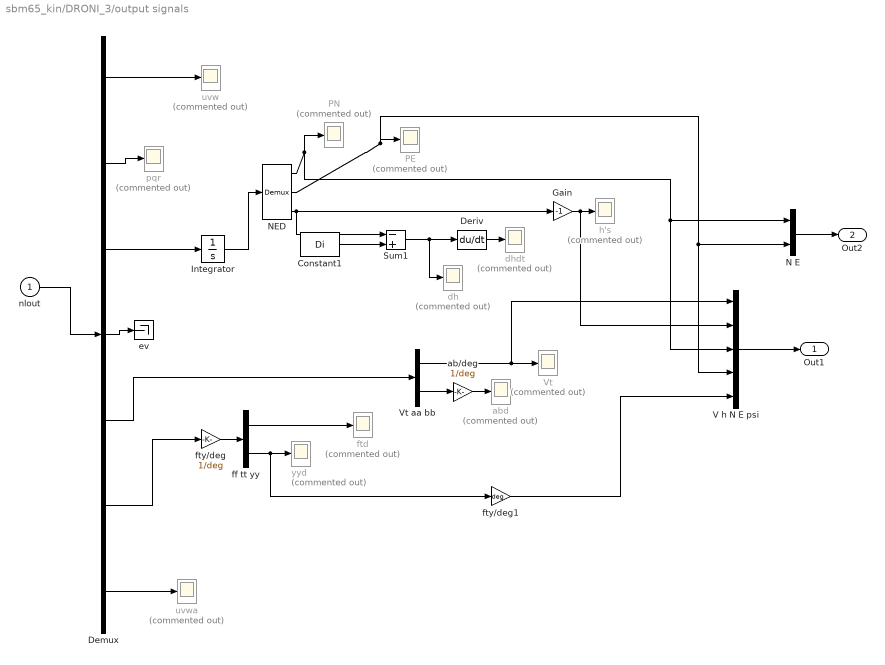
== system sbm65_kin/DRONI_3/output signals ==
  nlout : Inport
  Constant1 : Constant  Value=Di
  Demux : Demux  Outputs=[3 3 3 4 3 3 3]
  Deriv : Derivative
  Gain : Gain  Gain=-1  SaturateOnIntegerOverflow=on  OutDataTypeStr=Inherit: Same as input  ParamDataTypeStr=Inherit: Same as input
  Integrator : Integrator  InitialCondition=X7_ini3(1:3)
  N E : Mux  Inputs=2
  NED : Demux  Outputs=3
  PE : Scope  Commented=on
  PN : Scope  Commented=on
  Sum1 : Sum  Inputs=-+  SaturateOnIntegerOverflow=on  InputSameDT=on  OutDataTypeStr=Inherit: Same as first input
  V h N E psi : Mux  Inputs=5
  Vt : Scope  Commented=on
  Vt aa bb : Demux  Outputs=[1 2]
  ab/deg : Gain  Gain=1/deg  SaturateOnIntegerOverflow=on  OutDataTypeStr=Inherit: Same as input  ParamDataTypeStr=Inherit: Same as input
  abd : Scope  Commented=on
  dh : Scope  Commented=on
  dhdt : Scope  Commented=on
  ev : Terminator
  ff tt yy : Demux  Outputs=[2 1]
  ftd : Scope  Commented=on
  fty/deg : Gain  Gain=1/deg  SaturateOnIntegerOverflow=on  OutDataTypeStr=Inherit: Same as input  ParamDataTypeStr=Inherit: Same as input
  fty/deg1 : Gain  Gain=deg  SaturateOnIntegerOverflow=on  OutDataTypeStr=Inherit: Same as input  ParamDataTypeStr=Inherit: Same as input
  h's : Scope  Commented=on
  pqr : Scope  Commented=on
  uvw : Scope  Commented=on
  uvwa : Scope  Commented=on
  yyd : Scope  Commented=on
  Out1 : Outport
  Out2 : Outport  Port=2
  wires:
  fty/deg/1 -> ff tt yy/1
  ab/deg/1 -> abd/1
  NED/1 -> N E/1, V h N E psi/3, PN/1
  NED/2 -> N E/2, V h N E psi/4, PE/1
  Gain/1 -> V h N E psi/2, h's/1
  NED/3 -> Gain/1, Sum1/1
  Sum1/1 -> dh/1, Deriv/1
  Constant1/1 -> Sum1/2
  Demux/4 -> ev/1
  Vt aa bb/2 -> ab/deg/1
  Vt aa bb/1 -> V h N E psi/1, Vt/1
  nlout/1 -> Demux/1
  Demux/2 -> pqr/1
  ff tt yy/1 -> ftd/1
  ff tt yy/2 -> fty/deg1/1, yyd/1
  Deriv/1 -> dhdt/1
  Demux/1 -> uvw/1
  Demux/3 -> Integrator/1
  Demux/5 -> Vt aa bb/1
  Demux/6 -> fty/deg/1
  Demux/7 -> uvwa/1
  Integrator/1 -> NED/1
  fty/deg1/1 -> V h N E psi/5
  V h N E psi/1 -> Out1/1
  N E/1 -> Out2/1

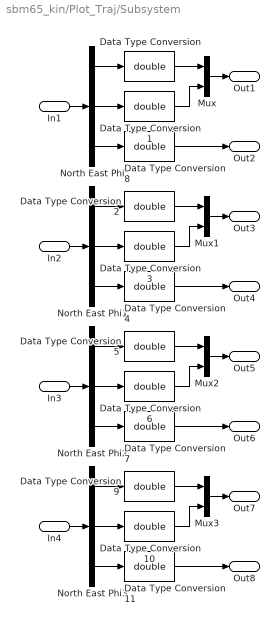
== system sbm65_kin/Plot_Traj/Subsystem ==
  In1 : Inport
  In2 : Inport  Port=2
  In3 : Inport  Port=3
  In4 : Inport  Port=4
  Data Type Conversion{,1..11} (12 alike) : DataTypeConversion  DisableCoverage=on  OutDataTypeStr=double
  Mux{,1..3} (4 alike) : Mux  Inputs=2
  North East Phi{,1..3} (4 alike) : Demux  Outputs=[1 1 1]
  Out1 : Outport
  Out2 : Outport  Port=2
  Out3 : Outport  Port=3
  Out4 : Outport  Port=4
  Out5 : Outport  Port=5
  Out6 : Outport  Port=6
  Out7 : Outport  Port=7
  Out8 : Outport  Port=8
  wires:
  In1/1 -> North East Phi/1
  Mux/1 -> Out1/1
  North East Phi/2 -> Data Type Conversion1/1
  Data Type Conversion1/1 -> Mux/2
  Data Type Conversion8/1 -> Out2/1
  North East Phi/3 -> Data Type Conversion8/1
  Data Type Conversion/1 -> Mux/1
  North East Phi/1 -> Data Type Conversion/1
  In2/1 -> North East Phi1/1
  Mux1/1 -> Out3/1
  North East Phi1/2 -> Data Type Conversion3/1
  Data Type Conversion3/1 -> Mux1/2
  Data Type Conversion4/1 -> Out4/1
  North East Phi1/3 -> Data Type Conversion4/1
  Data Type Conversion2/1 -> Mux1/1
  North East Phi1/1 -> Data Type Conversion2/1
  In3/1 -> North East Phi2/1
  Mux2/1 -> Out5/1
  North East Phi2/2 -> Data Type Conversion6/1
  Data Type Conversion6/1 -> Mux2/2
  Data Type Conversion7/1 -> Out6/1
  North East Phi2/3 -> Data Type Conversion7/1
  Data Type Conversion5/1 -> Mux2/1
  North East Phi2/1 -> Data Type Conversion5/1
  In4/1 -> North East Phi3/1
  Mux3/1 -> Out7/1
  North East Phi3/2 -> Data Type Conversion10/1
  Data Type Conversion10/1 -> Mux3/2
  Data Type Conversion11/1 -> Out8/1
  North East Phi3/3 -> Data Type Conversion11/1
  Data Type Conversion9/1 -> Mux3/1
  North East Phi3/1 -> Data Type Conversion9/1

== matlab function sbm65_kin/DRONI_2/MATLAB Function ==
  data: mis input; out output; distError input; simTime input
function out = misTracking(mis,distError,simTime)
% MISTRACKING
%
% Chooses point to be set as destination, according to mis matrix.

persistent misPointer timeOutStart hoverFlag;

if isempty(misPointer)
    misPointer = 1;    % initalize the persistent variable
end
if isempty(timeOutStart)
    timeOutStart = 0;  % initalize the persistent variable
end
if isempty(hoverFlag)  % 0 - no hover; 1 - moving to hover; 2 - hovering
    hoverFlag = 0;     % initalize the persistent variable
end

hoverTime = mis(misPointer,4);

if (hoverTime ~= 0 && hoverFlag == 0)
    hoverFlag = 1;
end

if (hoverFlag == 0 && abs(distError) <= 2 && simTime - timeOutStart > 0.1)
    misPointer = misPointer + 1; % Changes objective if distance to target 
    timeOutStart = simTime;      % is less than 1 m
end        

% Hover settings
if (hoverFlag == 1 && abs(distError) <= 5 && simTime - timeOutStart > 0.1)
    timeOutStart = simTime;
    hoverFlag = 2;
elseif (hoverFlag == 2 && simTime - timeOutStart > hoverTime)
    misPointer = misPointer + 1;
    hoverFlag = 0;
    timeOutStart = simTime;
end

if misPointer > size(mis,1)         % Repeats mission
    misPointer = 1;
end

out = [mis(misPointer,1:3), hoverFlag];

== matlab function sbm65_kin/DRONI_1/MATLAB Function ==
  data: mis input; out output; distError input; simTime input
function out = misTracking(mis,distError,simTime)
% MISTRACKING
%
% Chooses point to be set as destination, according to mis matrix.

persistent misPointer timeOutStart hoverFlag;

if isempty(misPointer)
    misPointer = 1;    % initalize the persistent variable
end
if isempty(timeOutStart)
    timeOutStart = 0;  % initalize the persistent variable
end
if isempty(hoverFlag)  % 0 - no hover; 1 - moving to hover; 2 - hovering
    hoverFlag = 0;     % initalize the persistent variable
end

hoverTime = mis(misPointer,4);

if (hoverTime ~= 0 && hoverFlag == 0)
    hoverFlag = 1;
end

if (hoverFlag == 0 && abs(distError) <= 2 && simTime - timeOutStart > 0.1)
    misPointer = misPointer + 1; % Changes objective if distance to target 
    timeOutStart = simTime;      % is less than 1 m
end        

% Hover settings
if (hoverFlag == 1 && abs(distError) <= 5 && simTime - timeOutStart > 0.1)
    timeOutStart = simTime;
    hoverFlag = 2;
elseif (hoverFlag == 2 && simTime - timeOutStart > hoverTime)
    misPointer = misPointer + 1;
    hoverFlag = 0;
    timeOutStart = simTime;
end

if misPointer > size(mis,1)         % Repeats mission
    misPointer = 1;
end

out = [mis(misPointer,1:3), hoverFlag];

== matlab function sbm65_kin/DRONI_3/MATLAB Function ==
  data: mis input; out output; distError input; simTime input
function out = misTracking(mis,distError,simTime)
% MISTRACKING
%
% Chooses point to be set as destination, according to mis matrix.

persistent misPointer timeOutStart hoverFlag;

if isempty(misPointer)
    misPointer = 1;    % initalize the persistent variable
end
if isempty(timeOutStart)
    timeOutStart = 0;  % initalize the persistent variable
end
if isempty(hoverFlag)  % 0 - no hover; 1 - moving to hover; 2 - hovering
    hoverFlag = 0;     % initalize the persistent variable
end

hoverTime = mis(misPointer,4);

if (hoverTime ~= 0 && hoverFlag == 0)
    hoverFlag = 1;
end

if (hoverFlag == 0 && abs(distError) <= 2 && simTime - timeOutStart > 0.1)
    misPointer = misPointer + 1; % Changes objective if distance to target 
    timeOutStart = simTime;      % is less than 1 m
end        

% Hover settings
if (hoverFlag == 1 && abs(distError) <= 5 && simTime - timeOutStart > 0.1)
    timeOutStart = simTime;
    hoverFlag = 2;
elseif (hoverFlag == 2 && simTime - timeOutStart > hoverTime)
    misPointer = misPointer + 1;
    hoverFlag = 0;
    timeOutStart = simTime;
end

if misPointer > size(mis,1)         % Repeats mission
    misPointer = 1;
end

out = [mis(misPointer,1:3), hoverFlag];

== matlab function sbm65_kin/Moving target ==
  data: t input; tar output
function tar = target(t)

min_v = 4;
max_v = 4;
min_w = -pi/10;
max_w = pi/10;
init_target = [0 0 3*pi/2];
persistent flag t_ state

if(isempty(flag))
    flag = 1;
    t_   = t;
    state = zeros(1,4);    
    state(1:2) = init_target(1:2);
    state(3)   = init_target(3);
    state(4)   = 0;
else
    dt = t-t_;
    
    % f function
    v = (max_v-min_v)*rand(1,1)+min_v;   
    if(randi(50,1,1)==20)
        w = (max_w-min_w)*rand(1,1)+min_w;
    else
        w=0;
    end
    u=[w,v];
    
    % command function
    x_=u(2)*cos(state(3));
    y_=u(2)*sin(state(3));
    theta_=u(1);
    v_=u(2);
    x_dot=[x_,y_,theta_,v_];
    
    state = state + [dt,dt,1,dt].*x_dot;
    t_ = t;
end

tar = zeros(1,3);
tar(1) = state(2);
tar(2) = state(1);
tar(3) = state(3);

end
